simulink model "RC_control_test"  (R2023b)
settings: Solver=ode4  StartTime=0.0  StopTime=inf  FixedStep=0.001  RelTol=1e-3
libraries: vrlib x1, aerolibanimutils x1
settings Model: Creator=admin  LastModifiedBy=ADMIN

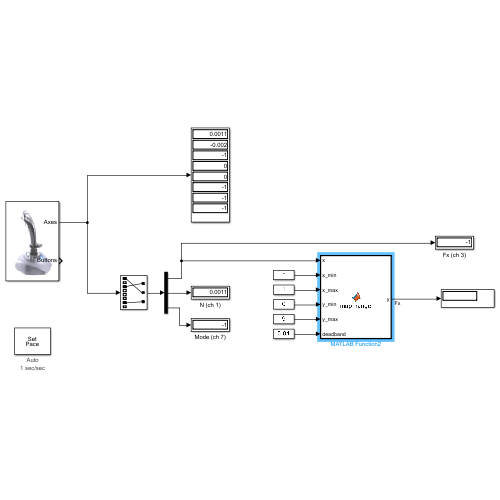
[thumbnail: Simulink's stored preview of the top-level diagram]
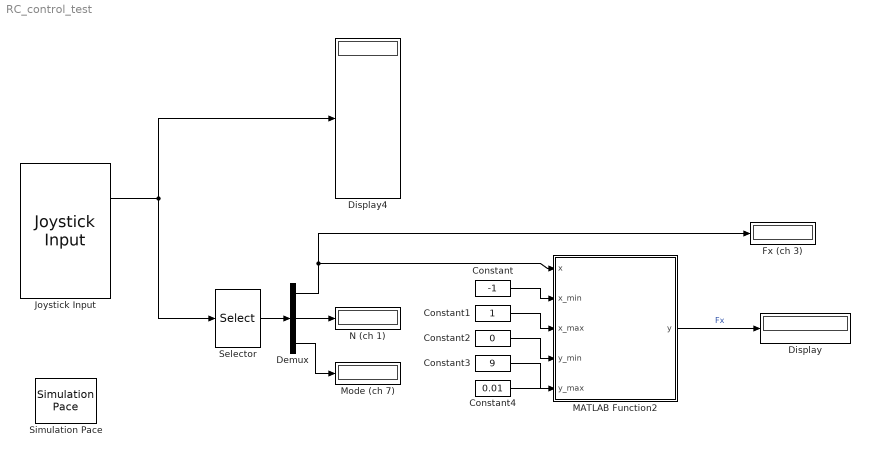
== system RC_control_test ==
  Constant : Constant  Value=-1
  Constant1 : Constant
  Constant2 : Constant  Value=0
  Constant3 : Constant  Value=9
  Constant4 : Constant  Value=0.01
  Demux : Demux  Outputs=3
  Display : Display
  Display4 : Display
  Fx (ch 3) : Display
  Joystick Input : vrlib/Joystick Input  joyid=1  adjustports=on  forcefeed=off
  MATLAB Function2 : MATLAB Function  TreatAsAtomicUnit=on
  Mode (ch 7) : Display
  N (ch 1) : Display
  Selector : Selector  InputPortWidth=8  IndexOptions=Index vector (dialog)  Indices=[3 1 7]  OutputSizes=1
  Simulation Pace : aerolibanimutils/Simulation Pace  SimulationPace=1  SleepMode=Auto  OutputPaceError=off  SampleTime=0.1
  wires:
  Joystick Input/1 -> Selector/1, Display4/1
  Selector/1 -> Demux/1
  Demux/1 -> Fx (ch 3)/1, MATLAB Function2/1(x)
  Demux/2 -> N (ch 1)/1
  Demux/3 -> Mode (ch 7)/1
  Constant/1 -> MATLAB Function2/2(x_min)
  Constant1/1 -> MATLAB Function2/3(x_max)
  Constant2/1 -> MATLAB Function2/4(y_min)
  Constant3/1 -> MATLAB Function2/5(y_max)
  MATLAB Function2/1(y) -> Display/1  "Fx"
  Constant4/1 -> ?

== matlab function RC_control_test/MATLAB Function2 ==
  data: x input; y output; x_min input; x_max input; y_min input; y_max input
% function y = map_range(x, x_min, x_max, y_min, y_max, deadband)
%     % 입력 범위 [x_min, x_max]를 출력 범위 [y_min, y_max]로 선형 매핑
%     % deadband: 입력 값이 [-deadband, deadband] 내에 있으면 출력 0
% 
%     y = zeros(size(x));  % 출력 초기화
% 
%     % deadband 바깥의 값만 선형 매핑 적용
%     mask = abs(x) > deadband;
%     y(mask) = (x(mask) - x_min) * (y_max - y_min) / (x_max - x_min) + y_min;
% end

function y = map_range(x, x_min, x_max, y_min, y_max)
    % 입력 범위 [x_min, x_max]를 출력 범위 [y_min, y_max]로 선형 매핑
    % deadband: 입력 값이 [-deadband, deadband] 내에 있으면 출력 0

    y = zeros(size(x));  % 출력 초기화

    % deadband 바깥의 값만 선형 매핑 적용
    y = (x - x_min) * (y_max - y_min) / (x_max - x_min) + y_min;
end
